simulink model "Subsystem"  (R2020b)
settings: Solver=VariableStepAuto  StartTime=0.0  StopTime=10.0  RelTol=1e-3
settings Model: Creator=Admin  LastModifiedBy=Admin
settings DataIOCC: SaveOutput=off  SaveTime=off

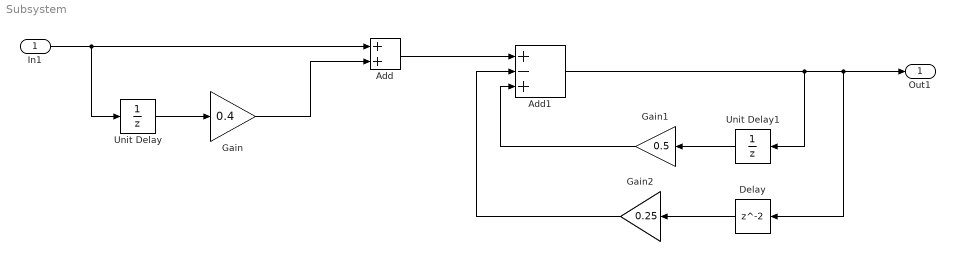
== system Subsystem ==
  In1 : Inport  OutDataTypeStr=double  PortDimensions=1  SampleTime=[0,1]
  Add : Sum
  Add1 : Sum  Inputs=+-+
  Delay : Delay
  Gain : Gain  Gain=0.4
  Gain1 : Gain  Gain=0.5
  Gain2 : Gain  Gain=0.25
  Unit Delay : UnitDelay  SampleTime=-1  HasFrameUpgradeWarning=on
  Unit Delay1 : UnitDelay  SampleTime=-1  HasFrameUpgradeWarning=on
  Out1 : Outport  OutDataTypeStr=double  PortDimensions=1  SampleTime=[0,1]
  wires:
  In1/1 -> Add/1, Unit Delay/1
  Add/1 -> Add1/1
  Unit Delay1/1 -> Gain1/1
  Gain/1 -> Add/2
  Gain2/1 -> Add1/2
  Unit Delay/1 -> Gain/1
  Gain1/1 -> Add1/3
  Delay/1 -> Gain2/1
  Add1/1 -> Delay/1, Out1/1, Unit Delay1/1
